simulink model "Sistema_camera_clean"  (R2015a)
settings: Solver=FixedStepDiscrete  StartTime=0.0  StopTime=12  FixedStep=.03  RelTol=1e-3
libraries: simulink x2, dspvision x1
settings Model: Creator=vmaraccini  LastModifiedBy=Administrator

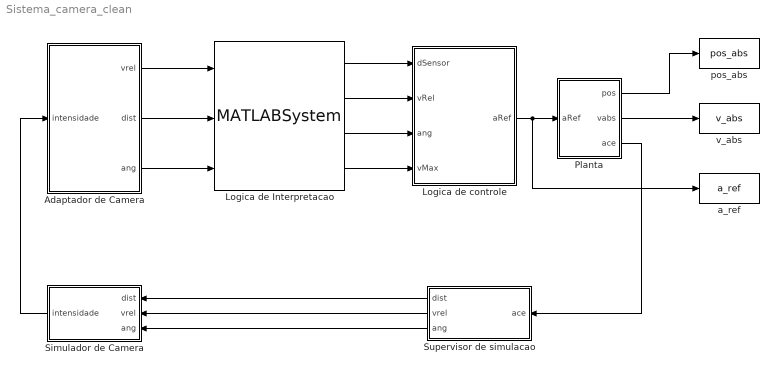
== system Sistema_camera_clean ==
  Adaptador de Camera : Subsystem
  Logica de Interpretacao : MATLABSystem  System=Interpretacao  SimulateUsing=Interpreted execution
      mask Type: Interpretacao
      mask Display:
      | disp('Interpretacao');
      | port_label('input',1,'vrel');
      | port_label('input',2,'dist');
      | port_label('input',3,'ang');
      | port_label('output',1,'d');
      | port_label('output',2,'v');
      | port_label('output',3,'a');
      | port_label('output',4,'max');
  Logica de controle : Subsystem
  Planta : Subsystem
  Simulador de Camera : Subsystem
  Supervisor de simulacao : Subsystem
  a_ref : ToWorkspace  VariableName=a_ref  SaveFormat=Timeseries  SampleTime=-1
  pos_abs : ToWorkspace  VariableName=pos_abs  SaveFormat=Timeseries  SampleTime=-1
  v_abs : ToWorkspace  VariableName=v_abs  SaveFormat=Timeseries  SampleTime=-1
  wires:
  Supervisor de simulacao/1(dist) -> Simulador de Camera/1(dist)
  Planta/3(ace) -> Supervisor de simulacao/1(ace)
  Planta/2(vabs) -> v_abs/1
  Supervisor de simulacao/3(ang) -> Simulador de Camera/3(ang)
  Supervisor de simulacao/2(vrel) -> Simulador de Camera/2(vrel)
  Logica de Interpretacao/1 -> Logica de controle/1(dSensor)
  Logica de controle/1(aRef) -> a_ref/1, Planta/1(aRef)
  Planta/1(pos) -> pos_abs/1
  Adaptador de Camera/1(vrel) -> Logica de Interpretacao/1
  Adaptador de Camera/2(dist) -> Logica de Interpretacao/2
  Adaptador de Camera/3(ang) -> Logica de Interpretacao/3
  Logica de Interpretacao/2 -> Logica de controle/2(vRel)
  Logica de Interpretacao/3 -> Logica de controle/3(ang)
  Logica de Interpretacao/4 -> Logica de controle/4(vMax)
  Simulador de Camera/1(intensidade) -> Adaptador de Camera/1(intensidade)

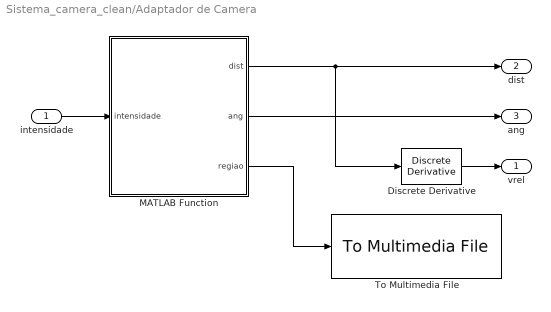
== system Sistema_camera_clean/Adaptador de Camera ==
  intensidade : Inport
  Discrete Derivative : simulink/Discrete/Discrete Derivative  gainval=1.0  ICPrevScaledInput=0.0  InputProcessing=Inherited  OutMin=[]  OutMax=[]  OutDataType=fixdt(1, 16)  OutScaling=2^-10  RndMeth=Ceiling  DoSatur=off
  MATLAB Function : MATLAB Function  TreatAsAtomicUnit=on
  To Multimedia File : dspvision/To Multimedia File  outputFilename=output_region.avi  streamSelection=Video only  videoCompressor=None (uncompressed)  audioCompressor=None (uncompressed)  imagePorts=One multidimensional signal  fileType=AVI  audioDatatype=Determine from input data type  fourcc=RGB  videoQuality=75  mj2000CompFactor=10
  vrel : Outport
  dist : Outport  Port=2
  ang : Outport  Port=3
  wires:
  intensidade/1 -> MATLAB Function/1(intensidade)
  MATLAB Function/2(ang) -> ang/1
  Discrete Derivative/1 -> vrel/1
  MATLAB Function/3(regiao) -> To Multimedia File/1
  MATLAB Function/1(dist) -> Discrete Derivative/1, dist/1

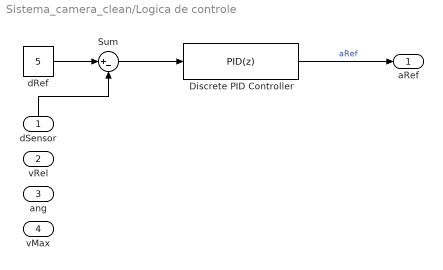
== system Sistema_camera_clean/Logica de controle ==
  dSensor : Inport
  vRel : Inport  Port=2
  ang : Inport  Port=3
  vMax : Inport  Port=4
  Discrete PID Controller : simulink/Continuous/PID Controller  Controller=PID  TimeDomain=Discrete-time  SampleTime=.03  IntegratorMethod=Forward Euler  FilterMethod=Forward Euler  Form=Parallel  UseFilter=on  ControllerParametersSource=internal  P=-1  I=0  D=-2  N=20  InitialConditionSource=internal  InitialConditionForIntegrator=0  InitialConditionForFilter=0  ExternalReset=none  LimitOutput=off  UpperSaturationLimit=5  LowerSaturationLimit=-2  LinearizeAsGain=off  AntiWindupMode=clamping  Kb=1  TrackingMode=off  Kt=1  PParamMin=[]  PParamMax=[]  IParamMin=[]  IParamMax=[]  DParamMin=[]  DParamMax=[]  NParamMin=[]  NParamMax=[]  KbParamMin=[]  KbParamMax=[]  KtParamMin=[]  KtParamMax=[]  POutMin=[]  POutMax=[]  IOutMin=[]  IOutMax=[]  DOutMin=[]  DOutMax=[]  NOutMin=[]  NOutMax=[]  KbOutMin=[]  KbOutMax=[]  KtOutMin=[]  KtOutMax=[]  IntegratorOutMin=[]  IntegratorOutMax=[]  FilterOutMin=[]  FilterOutMax=[]  SumOutMin=[]  SumOutMax=[]  SumI1OutMin=[]  SumI1OutMax=[]  SumI2OutMin=[]  SumI2OutMax=[]  SumI3OutMin=[]  SumI3OutMax=[]  SumDOutMin=[]  SumDOutMax=[]  SaturationOutMin=[]  SaturationOutMax=[]  IntegratorContinuousStateAttributes=''  IntegratorStateMustResolveToSignalObject=off  IntegratorRTWStateStorageClass=Auto  FilterContinuousStateAttributes=''  FilterStateMustResolveToSignalObject=off  FilterRTWStateStorageClass=Auto  DifferentiatorICPrevScaledInput=0  DifferentiatorOutMin=[]  DifferentiatorOutMax=[]
  Sum : Sum  Inputs=|+-
  dRef : Constant  Value=5
  aRef : Outport
  wires:
  dSensor/1 -> Sum/2
  Sum/1 -> Discrete PID Controller/1
  dRef/1 -> Sum/1
  Discrete PID Controller/1 -> aRef/1  "aRef"

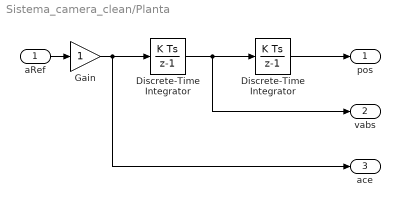
== system Sistema_camera_clean/Planta ==
  aRef : Inport
  Discrete-Time Integrator : DiscreteIntegrator  InitialConditionSetting=State (most efficient)  SampleTime=-1  StateIdentifier=posicao
  "Discrete-Time Integrator " : DiscreteIntegrator  gainval=.2  InitialCondition=10  InitialConditionSetting=State (most efficient)  SampleTime=-1  StateIdentifier=velocidade
  Gain : Gain
  pos : Outport
  vabs : Outport  Port=2
  ace : Outport  Port=3
  wires:
  aRef/1 -> Gain/1
  Discrete-Time Integrator/1 -> pos/1
  "Discrete-Time Integrator "/1 -> Discrete-Time Integrator/1, vabs/1
  Gain/1 -> "Discrete-Time Integrator "/1, ace/1

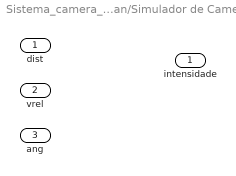
== system Sistema_camera_clean/Simulador de Camera ==
  dist : Inport
  vrel : Inport  Port=2
  ang : Inport  Port=3
  intensidade : Outport

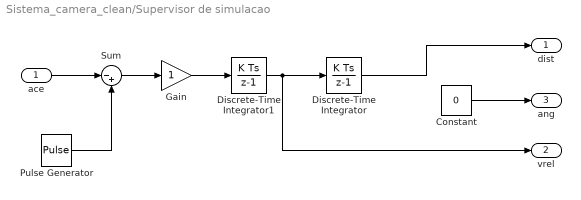
== system Sistema_camera_clean/Supervisor de simulacao ==
  ace : Inport  PortDimensions=1
  Constant : Constant  Value=0
  Discrete-Time Integrator : DiscreteIntegrator  InitialCondition=5  InitialConditionSetting=State (most efficient)  SampleTime=.03
  Discrete-Time Integrator1 : DiscreteIntegrator  InitialConditionSetting=State (most efficient)  SampleTime=.03
  Gain : Gain
  Pulse Generator : DiscretePulseGenerator  Amplitude=-3  Period=10000  PulseWidth=70  PhaseDelay=70  SampleTime=.03
  Sum : Sum  Inputs=|-+
  dist : Outport
  vrel : Outport  Port=2
  ang : Outport  Port=3
  wires:
  Discrete-Time Integrator1/1 -> Discrete-Time Integrator/1, vrel/1
  Sum/1 -> Gain/1
  Constant/1 -> ang/1
  Pulse Generator/1 -> Sum/2
  Discrete-Time Integrator/1 -> dist/1
  Gain/1 -> Discrete-Time Integrator1/1
  ace/1 -> Sum/1

== matlab function Sistema_camera_clean/Adaptador de Camera/MATLAB Function ==
  data: intensidade input; dist output; ang output; regiao output
function [dist,ang,regiao] = Adaptador_camera(intensidade)

width = length(intensidade(1,:));
height = length(intensidade(:,1));

hRange = floor(height*.5):ceil(height*.7);
wRange = floor(width*.45):ceil(width*.55);

regiao = intensidade(hRange, wRange);
average = mean(mean(regiao)); %Media da media das colunas

dist = 2*(1 - average);
ang = 0;

end
